simulink model "sampleModel1831_4_sub"  (R2023a)
settings: Solver=VariableStepAuto  StartTime=0.0  StopTime=10.0  RelTol=1e-3
libraries: hdlsllib x3, simulink x1
settings Model: Creator=user1  LastModifiedBy=user1
settings OptimizationCC: BlockReduction=off  ConditionallyExecuteInputs=off

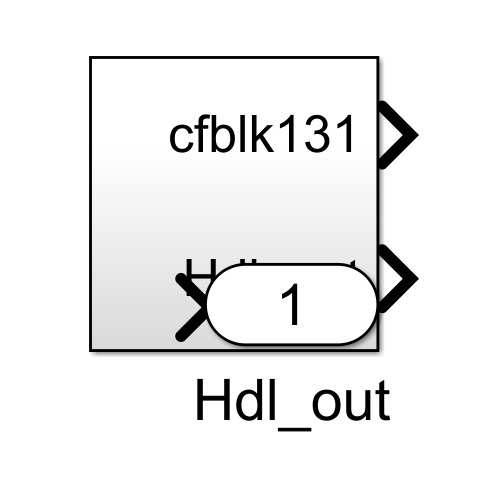
[thumbnail: Simulink's stored preview of the top-level diagram]
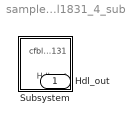
== system sampleModel1831_4_sub ==
  Subsystem : Subsystem
  Hdl_out : Outport  OutDataTypeStr=uint8

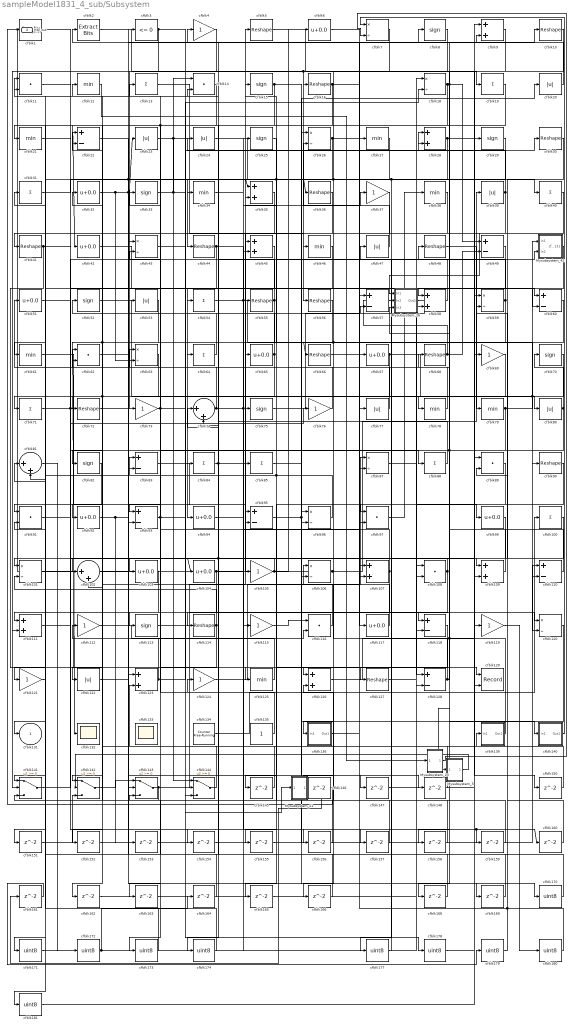
== system sampleModel1831_4_sub/Subsystem ==
  Mysubsystem_16 : Subsystem  TreatAsAtomicUnit=on  RTWFcnName=Mysubsystem_16
      settings: RTWFcnNameOpts=User specified  RTWFileNameOpts=Use function name
  Mysubsystem_21 : Subsystem  TreatAsAtomicUnit=on  RTWFcnName=Mysubsystem_21
      settings: RTWFcnNameOpts=User specified  RTWFileNameOpts=Use function name
  Mysubsystem_23 : Subsystem  TreatAsAtomicUnit=on  RTWFcnName=Mysubsystem_23
      settings: RTWFcnNameOpts=User specified  RTWFileNameOpts=Use function name
  Mysubsystem_42 : Subsystem  TreatAsAtomicUnit=on  RTWFcnName=Mysubsystem_42
      settings: RTWFcnNameOpts=User specified  RTWFileNameOpts=Use function name
  Mysubsystem_5 : Subsystem  TreatAsAtomicUnit=on  RTWFcnName=Mysubsystem_5
      settings: RTWFcnNameOpts=User specified  RTWFileNameOpts=Use function name
  cfblk1 : hdlsllib/Logic and Bit Operations/Detect Rise Nonnegative  vinit=0  OutDataTypeStr=uint8
  cfblk{5,10,16,30,36,41,44,48,55..56,66,68,72,90,114,127} (16 alike) : Reshape
  cfblk{13,19,31,40,54,64,71,84..85,88,100} (11 alike) : Sum  Inputs=+  OutDataTypeStr=uint8
  cfblk{7,18,26,43,59,63,87,96,101,106,120} (11 alike) : Product  Inputs=*/  OutDataTypeStr=uint8  RndMeth=Zero  SaturateOnIntegerOverflow=on
  cfblk102 : Sum  Inputs=|++  OutDataTypeStr=uint8
  cfblk{6,32,42,51,65,67,92,94,99,103..104,117} (12 alike) : Bias  Bias=0.0  SaturateOnIntegerOverflow=off
  cfblk{4,37,69,73,76,105,112,115,119,121,124} (11 alike) : Gain  OutDataTypeStr=uint8
  cfblk{9,28,35,45,58,107,109,111,123,126} (10 alike) : Sum  OutDataTypeStr=uint8
  cfblk{11,14,62,89,91,97,108,116} (8 alike) : DotProduct  OutDataTypeStr=uint8
  cfblk{22,49,57,60,83,93,95,110,118,128} (10 alike) : Sum  Inputs=+-  OutDataTypeStr=uint8
  cfblk{8,15,25,29,33,52,70,75,82,113} (10 alike) : Signum
  cfblk{12,21,27,34,38,46,61,78..79,125} (10 alike) : MinMax  OutDataTypeStr=uint8
  cfblk{20,23..24,39,47,53,77,80,122} (9 alike) : Abs  OutDataTypeStr=uint8  SaturateOnIntegerOverflow=off
  cfblk129 : Record  FileSettingsInternal="{\"entries\":[{\"content\":{\"excelSettings\":{\"content\":{},\"type\":\"Streamout.ExcelSettings\"}},\"type\":\"Streamout.FileSettingStorage\",\"uuid\":\"\"}],\"packageUris\":[\"http:\\/\\/schema.mathworks.com\\/mf0\\/streamout_blocks\\/R2020a\"],\"version\":\"1.0\"}"  Layout=[1 1]  SignalsInternal="{\"entries\":[{\"content\":{\"signals\":[{\"content\":{\"blockPath\":[],\"dimensions\":[1],\"domain\":\"\",\"lineColor\":\"#a2142f\",\"plots\":[1],\"port\":1,\"signalID\":44397,\"signalName\":\"cfblk41\"},\"type\":\"RecordBlkView.Signal\",\"uuid\":\"\"},{\"content\":{\"blockPath\":[],\"dimensions\":[1],\"domain\":\"\",\"lineColor\":\"#139fff\",\"plots\":[1],\"port\":2,\"signalID\":44400,\"signalName\":\"cfblk99\"},\"type\":\"RecordBlkView.Signal\",\"uuid\":\"\"}]},\"type\":\"RecordBlkView.InputSignals\",\"uuid\":\"\"}],\"packageUris\":[\"http:\\/\\/schema.mathworks.com\\/mf0\\/streamout_blocks\\/R2020a\"],\"version\":\"1.0\"}"  VisualizationBindings="{\"xyplotplugin\":{\"info\":[{\"series\":[{\"bindingParametersList\":[{\"parameter\":\"X-Axis\",\"signalID\":44397,\"signalName\":\"cfblk41\"},{\"parameter\":\"Y-Axis\",\"signalID\":44400,\"signalName\":\"cfblk99\"}],\"seriesID\":20981}],\"subplotID\":1}]}}"  CompatibilityTag=XY  st=-1
  cfblk132 : Scope
  cfblk133 : Scope
      settings: Floating=on
  cfblk134 : hdlsllib/Sources/Counter Free-Running  NumBits=16  tsamp=-1
  cfblk135 : Constant  OutDataTypeStr=uint8  SampleTime=-1
  cfblk136 : Subsystem
      settings: LibrarySourceBlock=|
      | hdlsllib/Ports &
      | Subsystems/Subsystem
  cfblk139 : Subsystem
      settings: LibrarySourceBlock=|
      | hdlsllib/Ports &
      | Subsystems/Subsystem
  cfblk140 : Subsystem
      settings: LibrarySourceBlock=|
      | hdlsllib/Ports &
      | Subsystems/Subsystem
  cfblk{141..144} (4 alike) : Switch  OutDataTypeStr=uint8  SaturateOnIntegerOverflow=off  InputSameDT=off
  cfblk{145..148,150..166,168..169} (23 alike) : Delay  SampleTime=1
  cfblk{170..174,177..181} (10 alike) : DataTypeConversion  OutDataTypeStr=uint8  SaturateOnIntegerOverflow=off  RndMeth=Floor
  cfblk2 : simulink/Logic and Bit Operations/Extract Bits  bitsToExtract=Upper half  numBits=8  bitIdxRange=[0 7]  outScalingMode=Preserve fixed-point scaling
      settings: LibrarySourceBlock=|
      | hdlsllib/Logic and Bit
      | Operations/Extract Bits
  cfblk3 : hdlsllib/Logic and Bit Operations/Compare To Zero  relop=<=  OutDataTypeStr=uint8
  cfblk74 : Sum  Inputs=|++  OutDataTypeStr=uint8
  cfblk81 : Sum  Inputs=|++  OutDataTypeStr=uint8
  cfblk131 : Outport  OutDataTypeStr=uint8  VectorParamsAs1DForOutWhenUnconnected=off
  Hdl_out : Outport  Port=2  OutDataTypeStr=uint8
  wires:
  cfblk97/1 -> cfblk38/1
  cfblk71/1 -> cfblk109/2, cfblk88/1
  cfblk78/1 -> cfblk51/1
  cfblk115/1 -> cfblk116/1
  cfblk109/1 -> cfblk44/1
  cfblk41/1 -> cfblk83/2, cfblk129/1
  cfblk59/1 -> cfblk144/2, cfblk48/1
  cfblk33/1 -> cfblk18/2, cfblk14/1
  cfblk7/1 -> cfblk111/2, cfblk56/1
  cfblk136/1(Out1) -> cfblk67/1
  cfblk46/1 -> cfblk94/1
  cfblk140/1(Out1) -> cfblk7/1
  cfblk60/1 -> cfblk174/1, cfblk104/1
  cfblk4/1 -> cfblk73/1
  cfblk134/1 -> cfblk100/1
  cfblk81/1 -> cfblk172/1
  cfblk43/1 -> cfblk78/1
  cfblk63/1 -> cfblk152/1, cfblk141/1
  cfblk49/1 -> cfblk71/1
  cfblk143/1 -> cfblk141/3, cfblk5/1
  cfblk16/1 -> cfblk181/1, cfblk19/1
  cfblk40/1 -> cfblk105/1
  cfblk32/1 -> cfblk63/2, cfblk106/2, cfblk23/1
  cfblk22/1 -> cfblk169/1, cfblk35/1
  cfblk87/1 -> cfblk99/1
  cfblk38/1 -> cfblk41/1
  cfblk2/1 -> cfblk16/1
  cfblk53/1 -> cfblk82/1, cfblk132/1
  cfblk75/1 -> cfblk27/1
  cfblk65/1 -> cfblk114/1, cfblk52/1
  cfblk13/1 -> cfblk46/1
  cfblk66/1 -> cfblk10/1
  cfblk139/1(Out1) -> cfblk106/1, Mysubsystem_16/3(In3)
  cfblk61/1 -> cfblk95/1
  cfblk14/1 -> cfblk92/1
  cfblk57/1 -> cfblk128/1
  cfblk25/1 -> cfblk65/1
  cfblk3/1 -> cfblk178/1, cfblk141/2
  cfblk125/1 -> cfblk62/1
  cfblk67/1 -> cfblk120/2, cfblk91/1
  cfblk91/1 -> cfblk76/1
  cfblk35/1 -> cfblk72/1
  cfblk121/1 -> cfblk31/1
  cfblk105/1 -> cfblk6/1, cfblk103/1
  cfblk24/1 -> cfblk77/1
  cfblk128/1 -> cfblk68/1, cfblk47/1
  cfblk106/1 -> Hdl_out/1, cfblk39/1
  cfblk19/1 -> cfblk173/1, cfblk42/1
  cfblk84/1 -> cfblk120/1, cfblk4/1
  cfblk51/1 -> cfblk60/1
  cfblk103/1 -> cfblk142/1
  cfblk92/1 -> cfblk153/1, cfblk123/1
  cfblk10/1 -> cfblk126/1
  cfblk142/1 -> cfblk143/1
  cfblk28/1 -> cfblk151/1, cfblk150/1
  cfblk70/1 -> cfblk110/2, cfblk122/1
  cfblk64/1 -> cfblk12/1
  cfblk80/1 -> cfblk70/1, cfblk87/2, Mysubsystem_5/1(In1)
  cfblk55/1 -> cfblk14/2, cfblk64/1
  cfblk74/1 -> cfblk13/1, cfblk147/1, cfblk80/1
  cfblk34/1 -> cfblk25/1
  cfblk124/1 -> cfblk87/1
  cfblk47/1 -> cfblk26/2
  cfblk9/1 -> cfblk58/1
  cfblk94/1 -> cfblk30/1
  cfblk44/1 -> cfblk144/3, cfblk160/1, cfblk159/1
  cfblk99/1 -> cfblk129/2
  cfblk113/1 -> cfblk118/1
  cfblk48/1 -> cfblk79/1
  cfblk144/1 -> cfblk123/2
  cfblk127/1 -> cfblk18/1
  cfblk20/1 -> cfblk2/1
  cfblk76/1 -> cfblk22/1
  cfblk83/1 -> cfblk115/1
  cfblk45/1 -> cfblk74/2
  cfblk101/1 -> cfblk125/1
  cfblk52/1 -> cfblk117/1
  cfblk95/1 -> cfblk127/1, cfblk20/1
  cfblk88/1 -> cfblk11/1
  cfblk54/1 -> cfblk37/1, cfblk90/1
  cfblk73/1 -> cfblk113/1, cfblk75/1
  cfblk58/1 -> cfblk15/1
  cfblk102/1 -> cfblk3/1
  cfblk135/1 -> cfblk83/1
  cfblk72/1 -> cfblk9/2
  cfblk68/1 -> cfblk49/2, Mysubsystem_16/2(In2)
  cfblk116/1 -> cfblk63/1
  cfblk126/1 -> cfblk29/1
  cfblk18/1 -> cfblk21/1, cfblk158/1, cfblk49/1
  cfblk104/1 -> cfblk97/2, cfblk111/1
  cfblk117/1 -> cfblk32/1
  cfblk96/1 -> cfblk11/2, cfblk55/1
  cfblk79/1 -> cfblk93/1, Mysubsystem_42/1(In1)
  cfblk36/1 -> cfblk96/2
  cfblk8/1 -> cfblk36/1, cfblk166/1, cfblk66/1
  cfblk119/1 -> cfblk180/1
  cfblk15/1 -> cfblk140/1(In1), cfblk54/1
  cfblk123/1 -> cfblk112/1, cfblk28/1
  cfblk114/1 -> cfblk163/1, cfblk101/2
  cfblk112/1 -> cfblk116/2
  cfblk31/1 -> cfblk34/1
  cfblk30/1 -> cfblk109/1
  cfblk1/1 -> cfblk40/1
  cfblk26/1 -> cfblk28/2, cfblk84/1
  cfblk77/1 -> cfblk62/2
  cfblk23/1 -> cfblk144/1, cfblk59/1
  cfblk27/1 -> cfblk93/2, cfblk45/1
  cfblk62/1 -> cfblk53/1
  cfblk42/1 -> cfblk118/2
  cfblk69/1 -> cfblk136/1(In1)
  cfblk100/1 -> cfblk108/2
  cfblk39/1 -> cfblk24/1, Mysubsystem_16/1(In1)
  cfblk93/1 -> cfblk33/1, Mysubsystem_21/1(In1)
  cfblk107/1 -> cfblk155/1, cfblk43/2
  cfblk108/1 -> cfblk121/1, cfblk101/1
  cfblk5/1 -> cfblk69/1
  cfblk29/1 -> cfblk97/1, cfblk61/1
  cfblk6/1 -> cfblk60/2
  cfblk110/1 -> cfblk8/1
  cfblk56/1 -> cfblk102/1
  cfblk90/1 -> cfblk145/1
  cfblk145/1 -> cfblk22/2
  cfblk37/1 -> cfblk146/1
  cfblk146/1 -> cfblk1/1
  cfblk147/1 -> cfblk9/1
  cfblk122/1 -> cfblk148/1
  cfblk148/1 -> cfblk35/2
  cfblk150/1 -> cfblk74/1
  cfblk151/1 -> cfblk142/3
  cfblk152/1 -> cfblk26/1
  cfblk153/1 -> cfblk45/2
  cfblk11/1 -> cfblk154/1
  cfblk154/1 -> cfblk96/1
  cfblk155/1 -> cfblk110/1
  cfblk111/1 -> cfblk156/1
  cfblk156/1 -> cfblk143/2
  cfblk21/1 -> cfblk157/1
  cfblk157/1 -> cfblk126/2
  cfblk158/1 -> cfblk102/2
  cfblk159/1 -> cfblk95/2
  cfblk160/1 -> cfblk59/2
  cfblk162/1 -> cfblk107/2
  cfblk163/1 -> cfblk58/2
  cfblk164/1 -> cfblk43/1
  cfblk118/1 -> cfblk165/1
  cfblk165/1 -> cfblk128/2
  cfblk166/1 -> cfblk143/3
  cfblk120/1 -> cfblk168/1
  cfblk168/1 -> cfblk57/1
  cfblk169/1 -> cfblk91/2
  cfblk85/1 -> cfblk170/1
  cfblk170/1 -> cfblk124/1
  cfblk82/1 -> cfblk171/1
  cfblk171/1 -> cfblk85/1
  cfblk172/1 -> cfblk108/1, cfblk164/1
  cfblk173/1 -> cfblk81/1
  cfblk174/1 -> cfblk81/2
  cfblk89/1 -> cfblk177/1
  cfblk177/1 -> cfblk57/2
  cfblk178/1 -> cfblk89/1
  cfblk161/1 -> cfblk179/1
  cfblk179/1 -> cfblk89/2
  cfblk180/1 -> cfblk107/1, cfblk139/1(In1)
  cfblk181/1 -> cfblk119/1
  Mysubsystem_5/1(Out1) -> cfblk142/2
  Mysubsystem_16/1(Out1) -> cfblk162/1
  Mysubsystem_21/1(Out1) -> cfblk161/1
  cfblk12/1 -> Mysubsystem_23/1(In1)
  Mysubsystem_23/1(Out1) -> cfblk7/2
  cfblk141/1 -> Mysubsystem_42/2(In2)
  Mysubsystem_42/1(cfblk131) -> cfblk131/1

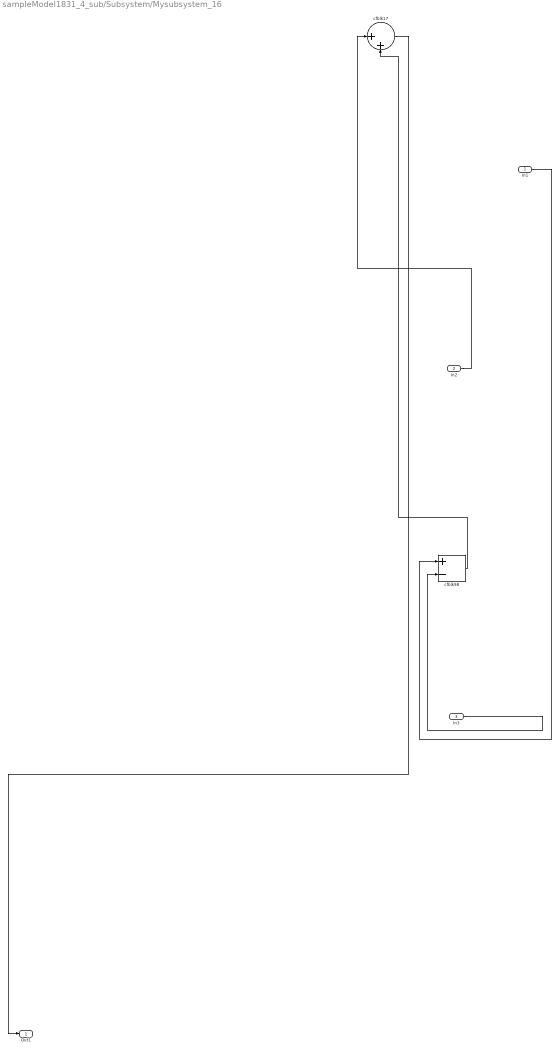
== system sampleModel1831_4_sub/Subsystem/Mysubsystem_16 ==
  In1 : Inport
  In2 : Inport  Port=2
  In3 : Inport  Port=3
  cfblk17 : Sum  Inputs=|++
  cfblk98 : Sum  Inputs=+-
  Out1 : Outport
  wires:
  cfblk17/1 -> Out1/1
  In1/1 -> cfblk98/1
  In2/1 -> cfblk17/1
  cfblk98/1 -> cfblk17/2
  In3/1 -> cfblk98/2

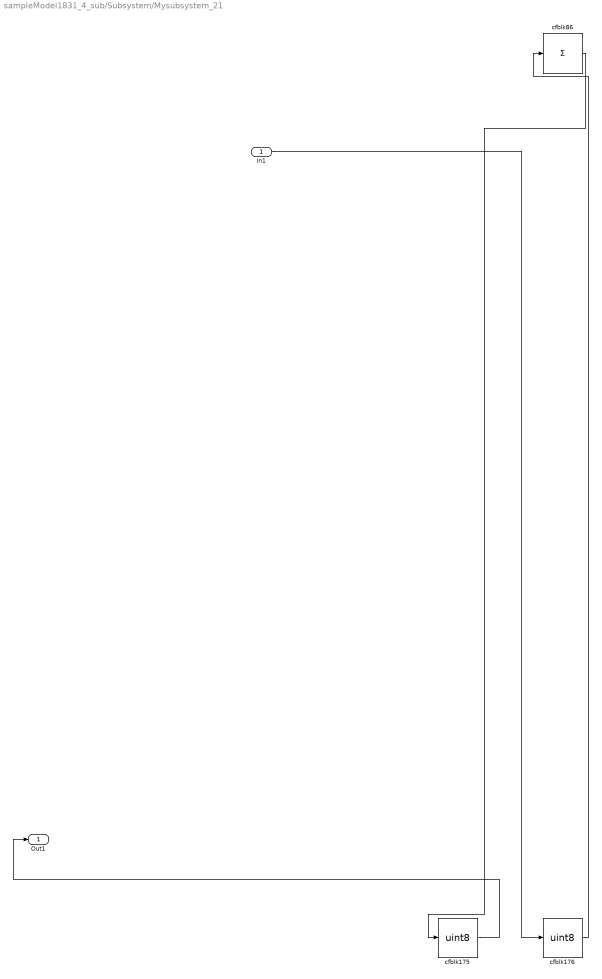
== system sampleModel1831_4_sub/Subsystem/Mysubsystem_21 ==
  In1 : Inport
  cfblk175 : DataTypeConversion  OutDataTypeStr=uint8  SaturateOnIntegerOverflow=off  RndMeth=Floor
  cfblk176 : DataTypeConversion  OutDataTypeStr=uint8  SaturateOnIntegerOverflow=off  RndMeth=Floor
  cfblk86 : Sum  Inputs=+
  Out1 : Outport
  wires:
  In1/1 -> cfblk176/1
  cfblk176/1 -> cfblk86/1
  cfblk175/1 -> Out1/1
  cfblk86/1 -> cfblk175/1

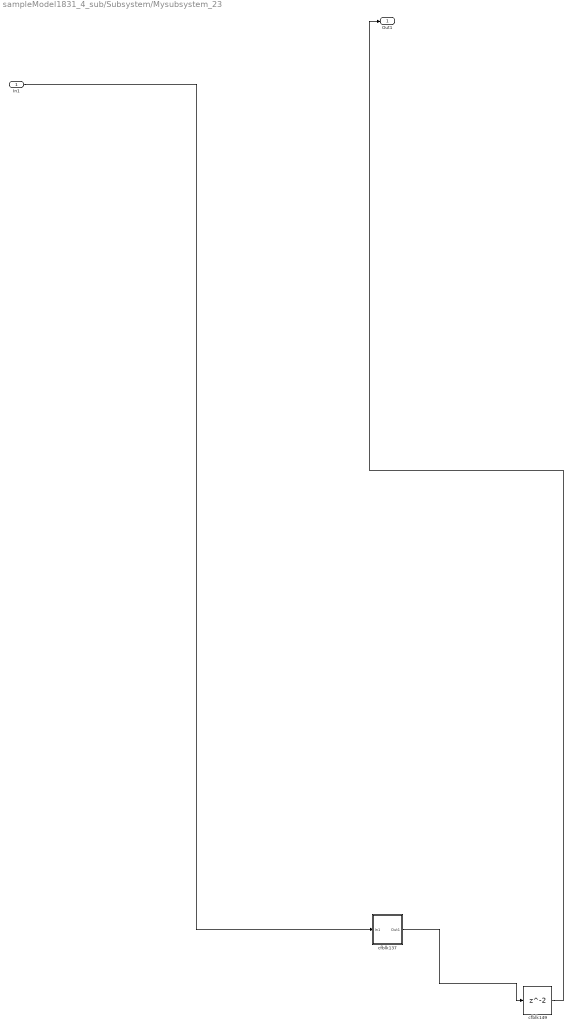
== system sampleModel1831_4_sub/Subsystem/Mysubsystem_23 ==
  In1 : Inport
  cfblk137 : Subsystem
      settings: LibrarySourceBlock=|
      | hdlsllib/Ports &
      | Subsystems/Subsystem
  cfblk149 : Delay  SampleTime=1
  Out1 : Outport
  wires:
  cfblk149/1 -> Out1/1
  cfblk137/1(Out1) -> cfblk149/1
  In1/1 -> cfblk137/1(In1)

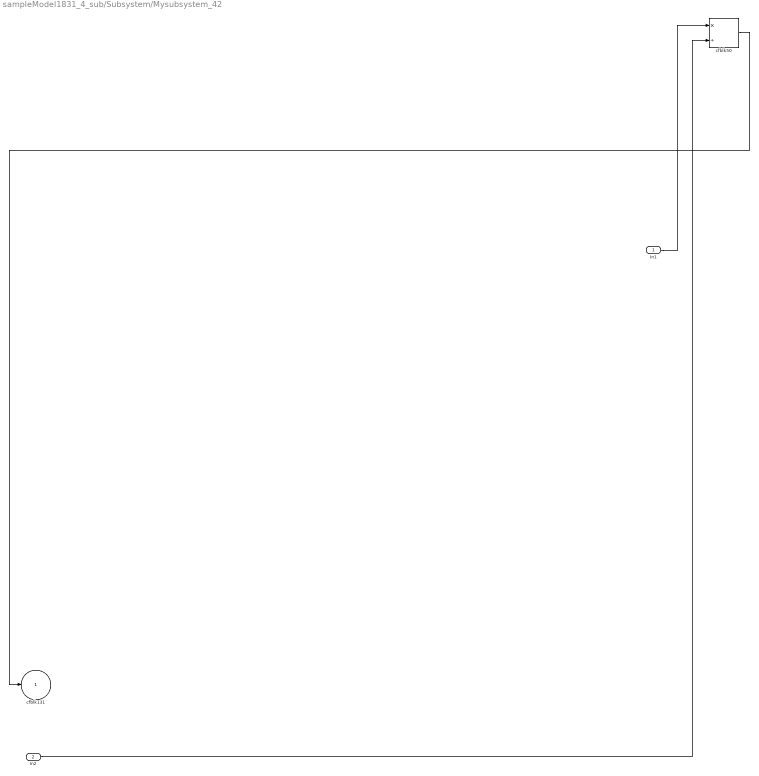
== system sampleModel1831_4_sub/Subsystem/Mysubsystem_42 ==
  In1 : Inport
  In2 : Inport  Port=2
  cfblk50 : Product  Inputs=*/  RndMeth=Zero  SaturateOnIntegerOverflow=on
  cfblk131 : Outport  VectorParamsAs1DForOutWhenUnconnected=off
  wires:
  In1/1 -> cfblk50/1
  In2/1 -> cfblk50/2
  cfblk50/1 -> cfblk131/1

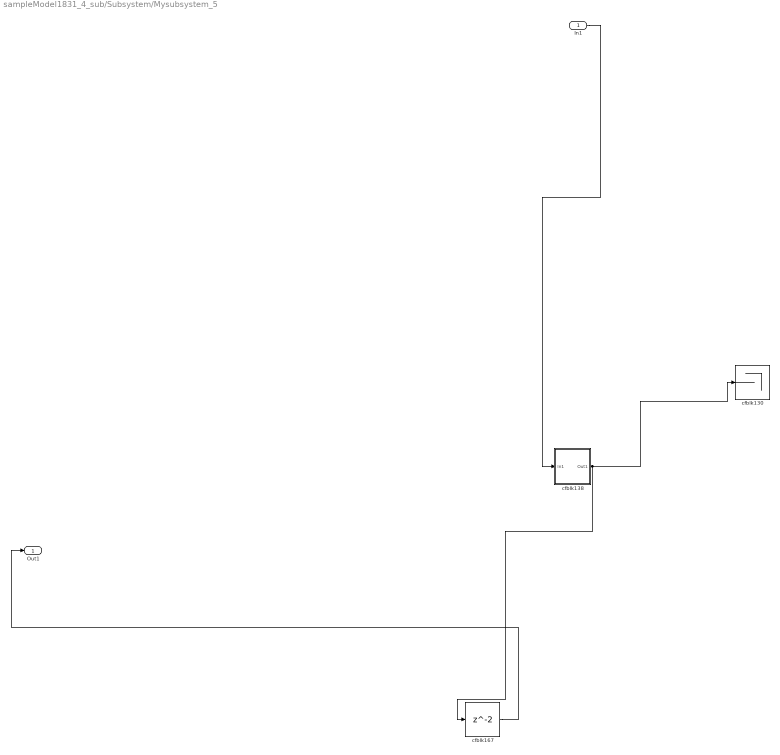
== system sampleModel1831_4_sub/Subsystem/Mysubsystem_5 ==
  In1 : Inport
  cfblk130 : Terminator
  cfblk138 : Subsystem
      settings: LibrarySourceBlock=|
      | hdlsllib/Ports &
      | Subsystems/Subsystem
  cfblk167 : Delay  SampleTime=1
  Out1 : Outport
  wires:
  cfblk167/1 -> Out1/1
  In1/1 -> cfblk138/1(In1)
  cfblk138/1(Out1) -> cfblk167/1, cfblk130/1

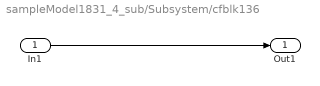
== system sampleModel1831_4_sub/Subsystem/cfblk136 ==
  In1 : Inport
  Out1 : Outport
  wires:
  In1/1 -> Out1/1

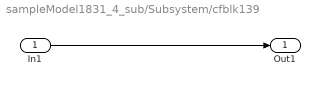
== system sampleModel1831_4_sub/Subsystem/cfblk139 ==
  In1 : Inport
  Out1 : Outport
  wires:
  In1/1 -> Out1/1

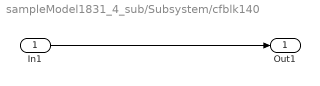
== system sampleModel1831_4_sub/Subsystem/cfblk140 ==
  In1 : Inport
  Out1 : Outport
  wires:
  In1/1 -> Out1/1

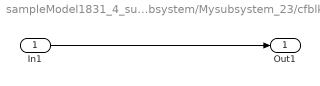
== system sampleModel1831_4_sub/Subsystem/Mysubsystem_23/cfblk137 ==
  In1 : Inport
  Out1 : Outport
  wires:
  In1/1 -> Out1/1

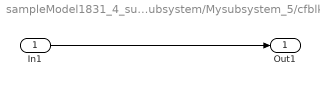
== system sampleModel1831_4_sub/Subsystem/Mysubsystem_5/cfblk138 ==
  In1 : Inport
  Out1 : Outport
  wires:
  In1/1 -> Out1/1
